simulink model "W04_P4_lowpass"  (R2024b)
settings: Solver=ode4  StartTime=0.0  StopTime=20  FixedStep=0.001  RelTol=1e-3
values from neighbouring files (symbols this model uses):
  lp_A_noise = 0.3    [W04_setup.m]
  lp_A_sig = 1.0    (= 1)    [W04_setup.m]
  lp_w_noise = 40    [W04_setup.m]
  lp_w_sig = 0.5    [W04_setup.m]
  lp_wc = 20    [W04_setup.m]
settings Model: Creator=admin  LastModifiedBy=admin

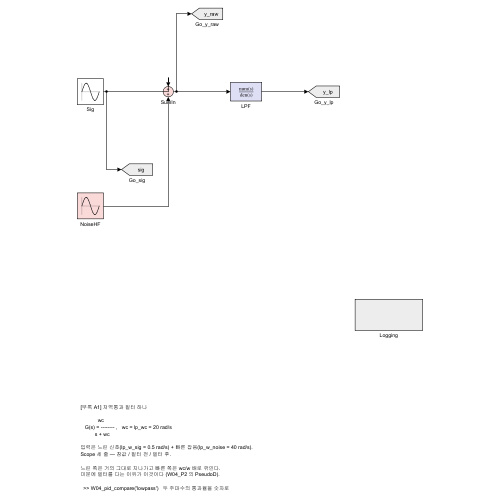
[thumbnail: Simulink's stored preview of the top-level diagram]
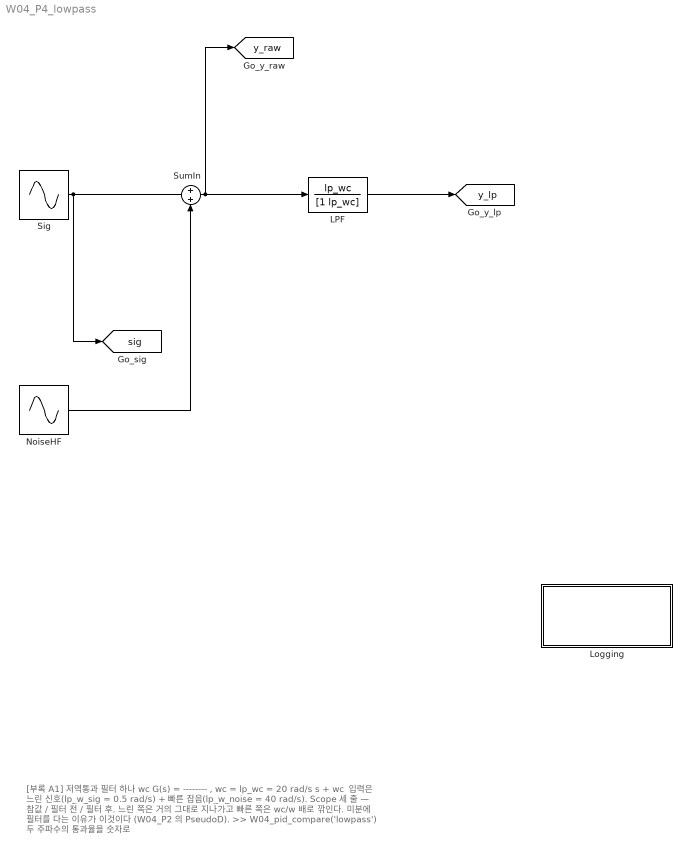
== system W04_P4_lowpass ==
  note: [부록 A1] 저역통과 필터 하나
      |
      |             wc
      |    G(s) = -------- ,   wc = lp_wc = 20 rad/s
      |           s + wc
      |
      | 입력은 느린 신호(lp_w_sig = 0.5 rad/s) + 빠른 잡음(lp_w_noise = 40 rad/s).
      | Scope 세 줄 — 참값 / 필터 전 / 필터 후.
      |
      | 느린 쪽은 거의 그대로 지나가고 빠른 쪽은 wc/w 배로 깎인다.
      | 미분에 필터를 다는 이유가 이것이다 (W04_P2 의 PseudoD).
      |
      |   >> W04_pid_compare('lowpass')   두 주파수의 통과율을 숫자로
  LPF : TransferFcn  Numerator=lp_wc  Denominator=[1 lp_wc]
  Logging : Subsystem
  NoiseHF : Sin  Amplitude=lp_A_noise  Frequency=lp_w_noise  SampleTime=0
  Sig : Sin  Amplitude=lp_A_sig  Frequency=lp_w_sig  SampleTime=0
  SumIn : Sum
  tag scope: sig=global, y_lp=global, y_raw=global
  wires:
  Sig/1 -> SumIn/1, [sig]
  NoiseHF/1 -> SumIn/2
  SumIn/1 -> LPF/1, [y_raw]
  LPF/1 -> [y_lp]

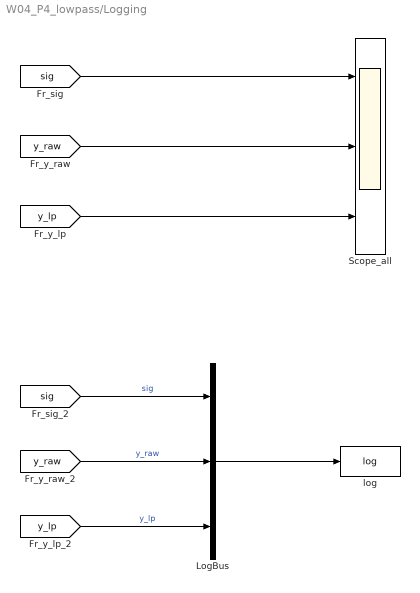
== system W04_P4_lowpass/Logging ==
  LogBus : BusCreator  Inputs=3
  Scope_all : Scope  NumInputPorts=3
  log : ToWorkspace  VariableName=log  SaveFormat=Timeseries  SampleTime=-1
  wires:
  [sig] -> Scope_all/1
  [y_raw] -> Scope_all/2
  [y_lp] -> Scope_all/3
  [sig] -> LogBus/1  "sig"
  [y_raw] -> LogBus/2  "y_raw"
  [y_lp] -> LogBus/3  "y_lp"
  LogBus/1 -> log/1
